simulink model "bd_ser_elect_cosim"  (Simulink 4.1.1)
settings: Solver=ode1  SolverMode=SingleTasking  StartTime=0.0  StopTime=max(cyc_mph(:,1))  FixedStep=1  MaxStep=1  RelTol=1e-3  AbsTol=1e-3
undefined symbols (not defined in the file): cs_lo_soc, cs_max_pwr, cs_max_pwr_fall_rate, cs_max_pwr_rise_rate, cs_min_pwr, ex_calc, fc_emis, fc_spd_scale, fc_trq_scale, time_step, vinf
libraries: lib_cosimulation x21, lib_controls x4, lib_wheel x2, lib_help x2, lib_transmission x2, simulink3 x1, lib_interactive x1, lib_drive_cycle x1, lib_exhaust x1, lib_fuel_converter x1, lib_vehicle x1
settings Model: LastModifiedBy=ssprik  SaveTime=off  SaveOutput=off  LimitDataPoints=off  UnconnectedLineMsg=none  RTWTemplateMakefile=grt_vc.tmf  ExtModeTrigMode=oneshot  ExtModeArmWhenConnect=off
settings Model: ModifiedComment=|
  | mokeefe -- Thu Apr 18 08:09:28 2002 -- Version 1.121
  | saving the model:
  | o "without the model browser open"
  | o with only top-level screen visible
  | o and with "fit to view" enabled
settings Model: ModifiedHistory=|
  | mokeefe -- Thu Apr 18 08:09:28 2002 -- Version 1.121
  | saving the model:
  | o "without the model browser open"
  | o with only top-level screen visible
  | o and with "fit to view" enabled

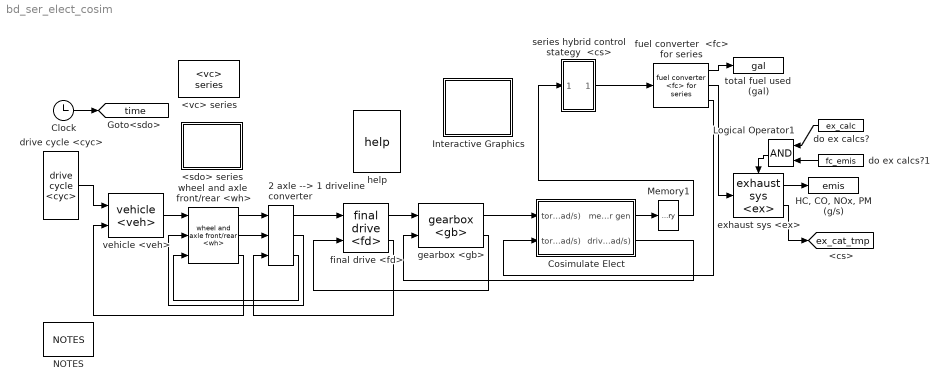
== system bd_ser_elect_cosim ==
  2 axle --> 1 driveline converter : lib_wheel/2 axle --> 1 driveline converter
      settings: RTWFcnNameOpts=Auto  RTWFileNameOpts=Auto
  <sdo> series : Subsystem
      settings: RTWFcnNameOpts=Auto  RTWFileNameOpts=Auto
      mask Display: image(imread('bdi_sdo.jpg'))
  <vc> series : lib_controls/<vc> series
      link override config traction control: BlockChoice=traction control
  Clock : Clock
      settings: DisplayTime=off  Decimation=10
  Cosimulate Elect : Subsystem  AncestorBlock=lib_cosimulation/SaberCosim
      settings: RTWFcnNameOpts=Auto  RTWFileNameOpts=Auto
      mask Display: image(imread('series_cosim.bmp'))
  "HC, CO, NOx, PM (g/s)" : ToWorkspace  VariableName=emis  SampleTime=0  SaveFormat=Array
  Interactive Graphics : Subsystem  BlockChoice=off
      link override off/Live Inputs/veh/roll res interactive: BlockChoice=roll res force req (N)
      settings: AttributesFormatString=%<BlockChoice>  TemplateBlock=lib_interactive/Interactive Graphics  MemberBlocks=off,on  RTWFcnNameOpts=Auto  RTWFileNameOpts=Auto
  Logical Operator1 : Logic  Orientation=left  Operator=AND  Inputs=2
  Memory1 : Memory  X0=0  InheritSampleTime=off
      settings: RTWStateStorageClass=Auto
  NOTES : lib_help/NOTES
  do ex calcs? : Constant  Orientation=left  Value=ex_calc
  do ex calcs?1 : Constant  Orientation=left  Value=fc_emis
  drive cycle <cyc> : lib_drive_cycle/drive cycle <cyc>
  exhaust sys <ex> : lib_exhaust/exhaust sys <ex>
  final drive <fd> : lib_transmission/final drive <fd>
  fuel converter  <fc> for series : lib_fuel_converter/fuel converter  <fc> for series
      link override fuel use and EO emis Configurable Subsystem: BlockChoice=fuel use and EO emis
  gearbox <gb> : lib_transmission/gearbox <gb>
  help : lib_help/help
  series hybrid control stategy  <cs> : Subsystem
      settings: RTWFcnNameOpts=Auto  RTWFileNameOpts=Auto
      mask Display: image(imread('bdi_cs.jpg'))
  total fuel used  (gal) : ToWorkspace  VariableName=gal  SampleTime=0  SaveFormat=Array
  vehicle <veh> : lib_vehicle/vehicle <veh>
      link override config force req'd to overcome rolling resistance: BlockChoice=force req'd to overcome rolling resistance (N)
      link override config vehicle speed: BlockChoice=vehicle speed (m/s)
      link override rolling resistance force: BlockChoice=force req'd to overcome rolling resistance (N)
      link override vehicle speed: BlockChoice=vehicle speed (m/s)
  wheel and axle  front/rear <wh> : lib_wheel/wheel and axle  front//rear <wh>
  tag scope: ex_cat_tmp=global, time=global
  wires:
  gearbox <gb>/1 -> Cosimulate Elect/1(torque and speed req'd at input side of gearbox (Nm),(rad/s))
  gearbox <gb>/2 -> final drive <fd>/2
  final drive <fd>/1 -> gearbox <gb>/1
  drive cycle <cyc>/1 -> vehicle <veh>/1
  Clock/1 -> [time]
  fuel converter  <fc> for series/2 -> exhaust sys <ex>/1
  fuel converter  <fc> for series/1 -> total fuel used  (gal)/1
  Logical Operator1/1 -> exhaust sys <ex>/Enable
  do ex calcs?/1 -> Logical Operator1/1
  exhaust sys <ex>/1 -> "HC, CO, NOx, PM (g/s)"/1
  do ex calcs?1/1 -> Logical Operator1/2
  exhaust sys <ex>/2 -> [ex_cat_tmp]
  fuel converter  <fc> for series/3 -> Cosimulate Elect/2(torque and speed available to drive line (Nm),(rad/s))
  Cosimulate Elect/2("drive torque and speed avail. at rotor (Nm), (rad/s)") -> gearbox <gb>/2
  Cosimulate Elect/1(mech pwr req'd for gen) -> Memory1/1
  Memory1/1 -> series hybrid control stategy  <cs>/1(mech power req'd from fc (W))
  series hybrid control stategy  <cs>/1("engine torque and speed (Nm), (rad/s)") -> fuel converter  <fc> for series/1
  vehicle <veh>/1 -> wheel and axle  front/rear <wh>/1
  wheel and axle  front/rear <wh>/1 -> 2 axle --> 1 driveline converter/1
  wheel and axle  front/rear <wh>/2 -> 2 axle --> 1 driveline converter/2
  2 axle --> 1 driveline converter/1 -> final drive <fd>/1
  2 axle --> 1 driveline converter/2 -> wheel and axle  front/rear <wh>/2
  2 axle --> 1 driveline converter/3 -> wheel and axle  front/rear <wh>/3
  final drive <fd>/2 -> 2 axle --> 1 driveline converter/3
  wheel and axle  front/rear <wh>/3 -> vehicle <veh>/2

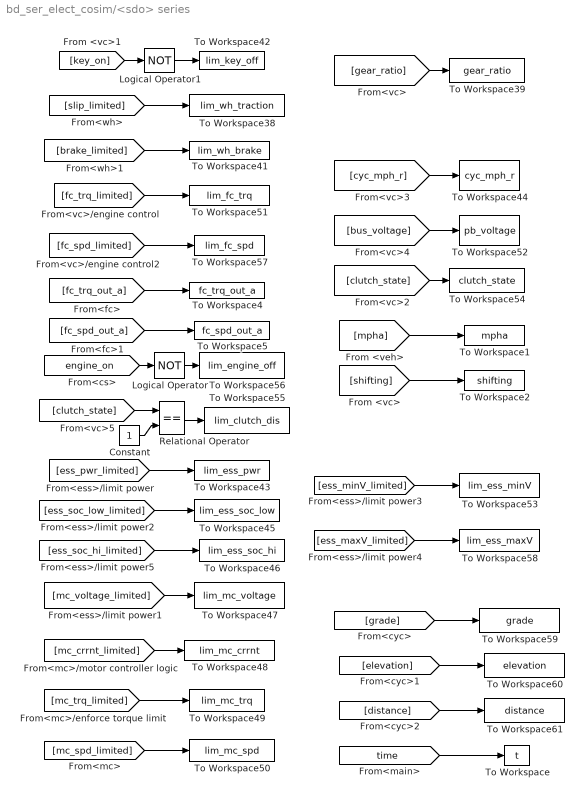
== system bd_ser_elect_cosim/<sdo> series ==
  Constant : Constant  Value=1
  Logical Operator : Logic  Operator=NOT  Inputs=1
  Logical Operator1 : Logic  Operator=NOT  Inputs=1
  Relational Operator : RelationalOperator  Operator===
  To Workspace : ToWorkspace  VariableName=t  SampleTime=0  SaveFormat=Array
  To Workspace1 : ToWorkspace  VariableName=mpha  SampleTime=-1  SaveFormat=Array
  To Workspace2 : ToWorkspace  VariableName=shifting  SampleTime=-1  SaveFormat=Array
  To Workspace38 : ToWorkspace  VariableName=lim_wh_traction  SampleTime=-1  SaveFormat=Array
  To Workspace39 : ToWorkspace  VariableName=gear_ratio  SampleTime=-1  SaveFormat=Array
  To Workspace4 : ToWorkspace  VariableName=fc_trq_out_a  SampleTime=-1  SaveFormat=Array
  To Workspace41 : ToWorkspace  VariableName=lim_wh_brake  SampleTime=-1  SaveFormat=Array
  To Workspace42 : ToWorkspace  VariableName=lim_key_off  SampleTime=-1  SaveFormat=Array
  To Workspace43 : ToWorkspace  VariableName=lim_ess_pwr  SampleTime=-1  SaveFormat=Array
  To Workspace44 : ToWorkspace  VariableName=cyc_mph_r  SampleTime=-1  SaveFormat=Array
  To Workspace45 : ToWorkspace  VariableName=lim_ess_soc_low  SampleTime=-1  SaveFormat=Array
  To Workspace46 : ToWorkspace  VariableName=lim_ess_soc_hi  SampleTime=-1  SaveFormat=Array
  To Workspace47 : ToWorkspace  VariableName=lim_mc_voltage  SampleTime=-1  SaveFormat=Array
  To Workspace48 : ToWorkspace  VariableName=lim_mc_crrnt  SampleTime=-1  SaveFormat=Array
  To Workspace49 : ToWorkspace  VariableName=lim_mc_trq  SampleTime=-1  SaveFormat=Array
  To Workspace5 : ToWorkspace  VariableName=fc_spd_out_a  SampleTime=-1  SaveFormat=Array
  To Workspace50 : ToWorkspace  VariableName=lim_mc_spd  SampleTime=-1  SaveFormat=Array
  To Workspace51 : ToWorkspace  VariableName=lim_fc_trq  SampleTime=-1  SaveFormat=Array
  To Workspace52 : ToWorkspace  VariableName=pb_voltage  SampleTime=-1  SaveFormat=Array
  To Workspace53 : ToWorkspace  VariableName=lim_ess_minV  SampleTime=-1  SaveFormat=Array
  To Workspace54 : ToWorkspace  VariableName=clutch_state  SampleTime=-1  SaveFormat=Array
  To Workspace55 : ToWorkspace  VariableName=lim_clutch_dis  SampleTime=-1  SaveFormat=Array
  To Workspace56 : ToWorkspace  VariableName=lim_engine_off  SampleTime=-1  SaveFormat=Array
  To Workspace57 : ToWorkspace  VariableName=lim_fc_spd  SampleTime=-1  SaveFormat=Array
  To Workspace58 : ToWorkspace  VariableName=lim_ess_maxV  SampleTime=-1  SaveFormat=Array
  To Workspace59 : ToWorkspace  VariableName=grade  SampleTime=-1  SaveFormat=Array
  To Workspace60 : ToWorkspace  VariableName=elevation  SampleTime=-1  SaveFormat=Array
  To Workspace61 : ToWorkspace  VariableName=distance  SampleTime=-1  SaveFormat=Array
  wires:
  [time] -> To Workspace/1
  [clutch_state] -> Relational Operator/1
  [fc_spd_out_a] -> To Workspace5/1
  [fc_trq_out_a] -> To Workspace4/1
  [mc_spd_limited] -> To Workspace50/1
  [mc_trq_limited] -> To Workspace49/1
  [mc_crrnt_limited] -> To Workspace48/1
  [mc_voltage_limited] -> To Workspace47/1
  [ess_soc_hi_limited] -> To Workspace46/1
  [ess_soc_low_limited] -> To Workspace45/1
  [ess_pwr_limited] -> To Workspace43/1
  Logical Operator/1 -> To Workspace56/1
  [engine_on] -> Logical Operator/1
  Constant/1 -> Relational Operator/2
  Relational Operator/1 -> To Workspace55/1
  [distance] -> To Workspace61/1
  [elevation] -> To Workspace60/1
  [grade] -> To Workspace59/1
  [ess_minV_limited] -> To Workspace53/1
  [ess_maxV_limited] -> To Workspace58/1
  Logical Operator1/1 -> To Workspace42/1
  [key_on] -> Logical Operator1/1
  [shifting] -> To Workspace2/1
  [mpha] -> To Workspace1/1
  [clutch_state] -> To Workspace54/1
  [bus_voltage] -> To Workspace52/1
  [cyc_mph_r] -> To Workspace44/1
  [gear_ratio] -> To Workspace39/1
  [slip_limited] -> To Workspace38/1
  [brake_limited] -> To Workspace41/1
  [fc_spd_limited] -> To Workspace57/1
  [fc_trq_limited] -> To Workspace51/1

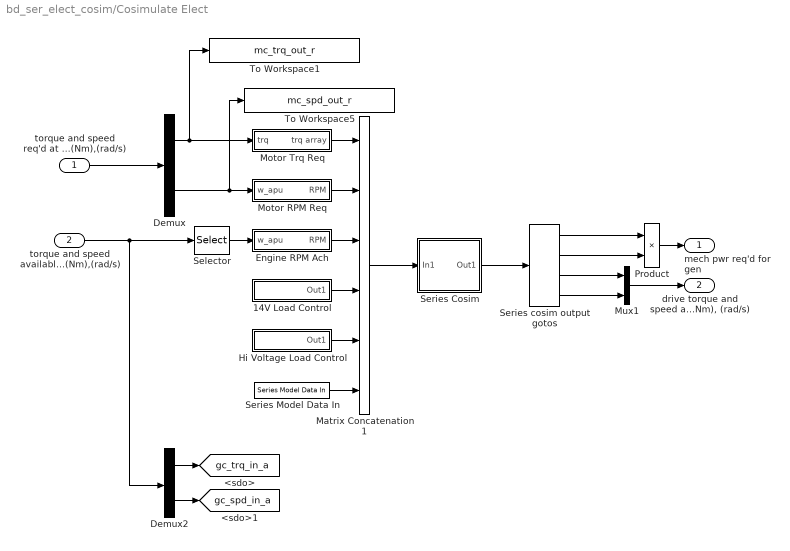
== system bd_ser_elect_cosim/Cosimulate Elect ==
  torque and speed req'd at input side of gearbox (Nm),(rad/s) : Inport  Port=1  LatchInput=off
  torque and speed available to drive line (Nm),(rad/s) : Inport  Port=2  LatchInput=off
  14V Load Control : Subsystem
      settings: RTWFcnNameOpts=Auto  RTWFileNameOpts=Auto
  Demux : Demux  Outputs=2  BusSelectionMode=off
  Demux2 : Demux  Outputs=2  BusSelectionMode=off
  Engine RPM Ach : Subsystem  AncestorBlock=lib_cosimulation/saber dv acc/Engine Info
      settings: RTWFcnNameOpts=Auto  RTWFileNameOpts=Auto
  Hi Voltage Load Control : Subsystem
      settings: RTWFcnNameOpts=Auto  RTWFileNameOpts=Auto
  Matrix Concatenation1 : simulink3/Signals & Systems/Matrix Concatenation  numInports=6  catMethod=Horizontal
  Motor RPM Req : Subsystem
      settings: RTWFcnNameOpts=Auto  RTWFileNameOpts=Auto
  Motor Trq Req : Subsystem
      settings: RTWFcnNameOpts=Auto  RTWFileNameOpts=Auto
  Mux1 : Mux  Inputs=2
  Product : Product  Inputs=2  Multiplication=Element-wise(.*)  SaturateOnIntegerOverflow=on
  Selector : Selector  InputType=Vector  ElementSrc=Internal  Elements=[2]  RowSrc=Internal  Rows=1  ColumnSrc=Internal  Columns=1  InputPortWidth=2
  Series Cosim : Subsystem  BlockChoice=Saber Text File Exchange
      settings: AttributesFormatString=%<BlockChoice>  TemplateBlock=lib_cosimulation/Series Cosim  MemberBlocks=Saber Text File Exchange,Series Saber Cosim,Series Simplorer Cosim  RTWFcnNameOpts=Auto  RTWFileNameOpts=Auto
  Series Model Data In : lib_cosimulation/Series Model Data In
  Series cosim output gotos : lib_cosimulation/Series cosim output gotos
      link override saber gc output gotos/Gain: Gain=1
      link override saber mc output gotos/sign convention: Gain=1
      settings: RTWFcnNameOpts=Auto  RTWFileNameOpts=Auto
  To Workspace1 : ToWorkspace  VariableName=mc_trq_out_r  SampleTime=-1  SaveFormat=Array
  To Workspace5 : ToWorkspace  VariableName=mc_spd_out_r  SampleTime=-1  SaveFormat=Array
  mech pwr req'd for gen : Outport  Port=1
  "drive torque and speed avail. at rotor (Nm), (rad/s)" : Outport  Port=2  InitialOutput=0
  tag scope: gc_spd_in_a=global, gc_trq_in_a=global
  wires:
  torque and speed req'd at input side of gearbox (Nm),(rad/s)/1 -> Demux/1
  Demux2/1 -> [gc_trq_in_a]
  Demux2/2 -> [gc_spd_in_a]
  Matrix Concatenation1/1 -> Series Cosim/1(In1)
  Series Cosim/1(Out1) -> Series cosim output gotos/1
  Mux1/1 -> "drive torque and speed avail. at rotor (Nm), (rad/s)"/1
  Series cosim output gotos/1 -> Product/1
  torque and speed available to drive line (Nm),(rad/s)/1 -> Selector/1, Demux2/1
  Demux/2 -> Motor RPM Req/1(w_apu), To Workspace5/1
  Motor RPM Req/1(RPM) -> Matrix Concatenation1/2
  Demux/1 -> Motor Trq Req/1(trq), To Workspace1/1
  Engine RPM Ach/1(RPM) -> Matrix Concatenation1/3
  Selector/1 -> Engine RPM Ach/1(w_apu)
  Motor Trq Req/1(trq array) -> Matrix Concatenation1/1
  Hi Voltage Load Control/1(Out1) -> Matrix Concatenation1/5
  14V Load Control/1(Out1) -> Matrix Concatenation1/4
  Series Model Data In/1 -> Matrix Concatenation1/6
  Series cosim output gotos/4 -> Mux1/2
  Series cosim output gotos/3 -> Mux1/1
  Series cosim output gotos/2 -> Product/2
  Product/1 -> mech pwr req'd for gen/1

== system bd_ser_elect_cosim/Interactive Graphics ==
  off : lib_interactive/off  Tag=Altia_off  Orientation=up

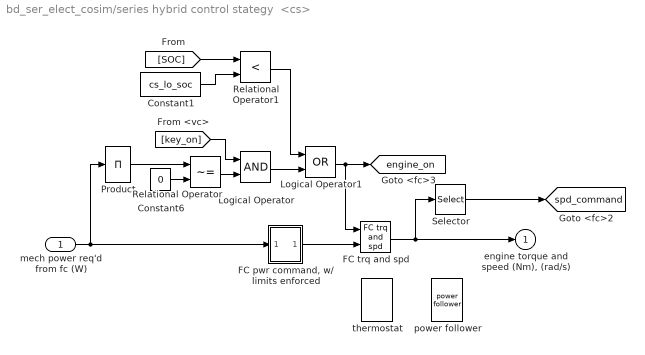
== system bd_ser_elect_cosim/series hybrid control stategy  <cs> ==
  mech power req'd from fc (W) : Inport  Port=1  LatchInput=off
  Constant1 : Constant  Value=cs_lo_soc
  Constant6 : Constant  Value=0
  "FC pwr command, w/ limits enforced" : Subsystem
      settings: RTWFcnNameOpts=Auto  RTWFileNameOpts=Auto
  FC trq and spd : lib_controls/series hybrid control stategy  <cs>/FC trq and spd
      settings: RTWFcnNameOpts=Auto  RTWFileNameOpts=Auto
  Logical Operator : Logic  Operator=AND  Inputs=2
  Logical Operator1 : Logic  Operator=OR  Inputs=2
  Product : Product  Inputs=1  Multiplication=Element-wise(.*)  SaturateOnIntegerOverflow=on
  Relational Operator : RelationalOperator  Operator=~=
  Relational Operator1 : RelationalOperator  Operator=<
  Selector : Selector  InputType=Vector  ElementSrc=Internal  Elements=2  RowSrc=Internal  Rows=1  ColumnSrc=Internal  Columns=1  InputPortWidth=2
  power follower : lib_controls/series hybrid control stategy  <cs>/power follower
  thermostat : lib_controls/series hybrid control stategy  <cs>/thermostat
  "engine torque and speed (Nm), (rad/s)" : Outport  Port=1  InitialOutput=0
  tag scope: engine_on=global, spd_command=global
  wires:
  Selector/1 -> [spd_command]
  mech power req'd from fc (W)/1 -> Product/1, "FC pwr command, w/ limits enforced"/1(FC pwr command)
  Constant6/1 -> Relational Operator/2
  Relational Operator/1 -> Logical Operator/2
  [key_on] -> Logical Operator/1
  Product/1 -> Relational Operator/1
  "FC pwr command, w/ limits enforced"/1(limited FC pwr command (W)) -> FC trq and spd/2
  FC trq and spd/1 -> "engine torque and speed (Nm), (rad/s)"/1, Selector/1
  Logical Operator1/1 -> [engine_on], FC trq and spd/1
  Logical Operator/1 -> Logical Operator1/2
  [SOC] -> Relational Operator1/1
  Constant1/1 -> Relational Operator1/2
  Relational Operator1/1 -> Logical Operator1/1

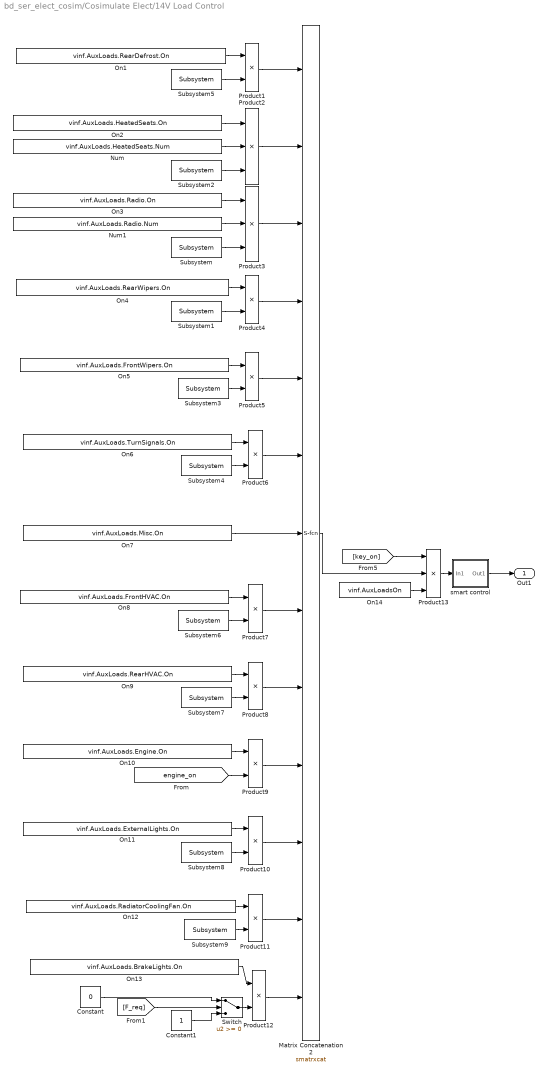
== system bd_ser_elect_cosim/Cosimulate Elect/14V Load Control ==
  Constant : Constant  Value=0
  Constant1 : Constant  Value=1
  Matrix Concatenation2 : S-Function  FunctionName=smatrxcat  Parameters=numInports,catMethod  PortCounts=[]  SFunctionModules=''  mask(Matrix Concatenation){numInports=13, catMethod=Horizontal}
      mask prompts: numInports "Number of inputs:"; catMethod "Concatenation method:"
      mask help: Perform horizontal or vertical concatenation. 1-D vector input signals are treated as column vectors, i.e., [Mx1] matrices. The output is always a matrix.
      mask init:
      | xy = matrxcatmask('icon');
      mask StyleString: edit,popup(Horizontal|Vertical)
      mask Display:
      | plot(xy.x,xy.y);
      | text(0.15,0.86,xy.label);
  Num : Constant  Value=vinf.AuxLoads.HeatedSeats.Num
  Num1 : Constant  Value=vinf.AuxLoads.Radio.Num
  On1 : Constant  Value=vinf.AuxLoads.RearDefrost.On
  On10 : Constant  Value=vinf.AuxLoads.Engine.On
  On11 : Constant  Value=vinf.AuxLoads.ExternalLights.On
  On12 : Constant  Value=vinf.AuxLoads.RadiatorCoolingFan.On
  On13 : Constant  Value=vinf.AuxLoads.BrakeLights.On
  On14 : Constant  Value=vinf.AuxLoadsOn
  On2 : Constant  Value=vinf.AuxLoads.HeatedSeats.On
  On3 : Constant  Value=vinf.AuxLoads.Radio.On
  On4 : Constant  Value=vinf.AuxLoads.RearWipers.On
  On5 : Constant  Value=vinf.AuxLoads.FrontWipers.On
  On6 : Constant  Value=vinf.AuxLoads.TurnSignals.On
  On7 : Constant  Value=vinf.AuxLoads.Misc.On
  On8 : Constant  Value=vinf.AuxLoads.FrontHVAC.On
  On9 : Constant  Value=vinf.AuxLoads.RearHVAC.On
  Product{1,4..12} (10 alike) : Product  Inputs=2  Multiplication=Element-wise(.*)  SaturateOnIntegerOverflow=on
  Product13 : Product  Inputs=3  Multiplication=Element-wise(.*)  SaturateOnIntegerOverflow=on
  Product2 : Product  Inputs=3  Multiplication=Element-wise(.*)  SaturateOnIntegerOverflow=on
  Product3 : Product  Inputs=3  Multiplication=Element-wise(.*)  SaturateOnIntegerOverflow=on
  Subsystem : lib_cosimulation/Subsystem  ModelName='Radio'
  Subsystem1 : lib_cosimulation/Subsystem  ModelName='RearWipers'
  Subsystem2 : lib_cosimulation/Subsystem  ModelName='HeatedSeats'
  Subsystem3 : lib_cosimulation/Subsystem  ModelName='FrontWipers'
  Subsystem4 : lib_cosimulation/Subsystem  ModelName='TurnSignals'
  Subsystem5 : lib_cosimulation/Subsystem  ModelName='RearDefrost'
  Subsystem6 : lib_cosimulation/Subsystem  ModelName='FrontHVAC'
  Subsystem7 : lib_cosimulation/Subsystem  ModelName='RearHVAC'
  Subsystem8 : lib_cosimulation/Subsystem  ModelName='ExternalLights'
  Subsystem9 : lib_cosimulation/Subsystem  ModelName='RadiatorCoolingFan'
  Switch : Switch  Threshold=0
  smart control : Subsystem
      settings: RTWFcnNameOpts=Auto  RTWFileNameOpts=Auto
  Out1 : Outport  Port=1
  wires:
  Subsystem/1 -> Product3/3
  Product1/1 -> Matrix Concatenation2/1
  smart control/1(Out1) -> Out1/1
  On14/1 -> Product13/3
  Subsystem5/1 -> Product1/2
  On1/1 -> Product1/1
  Subsystem2/1 -> Product2/3
  Num/1 -> Product2/2
  On2/1 -> Product2/1
  Num1/1 -> Product3/2
  On3/1 -> Product3/1
  Subsystem1/1 -> Product4/2
  On4/1 -> Product4/1
  Subsystem3/1 -> Product5/2
  On5/1 -> Product5/1
  On6/1 -> Product6/1
  Subsystem4/1 -> Product6/2
  On7/1 -> Matrix Concatenation2/7
  Subsystem6/1 -> Product7/2
  On8/1 -> Product7/1
  Subsystem7/1 -> Product8/2
  [engine_on] -> Product9/2
  On10/1 -> Product9/1
  Subsystem8/1 -> Product10/2
  On11/1 -> Product10/1
  Subsystem9/1 -> Product11/2
  On12/1 -> Product11/1
  Switch/1 -> Product12/2
  Constant1/1 -> Switch/3
  [F_req] -> Switch/2
  Constant/1 -> Switch/1
  On13/1 -> Product12/1
  Product2/1 -> Matrix Concatenation2/2
  Product3/1 -> Matrix Concatenation2/3
  Product4/1 -> Matrix Concatenation2/4
  Product5/1 -> Matrix Concatenation2/5
  Product6/1 -> Matrix Concatenation2/6
  Product7/1 -> Matrix Concatenation2/8
  Product8/1 -> Matrix Concatenation2/9
  Product9/1 -> Matrix Concatenation2/10
  Product10/1 -> Matrix Concatenation2/11
  Product11/1 -> Matrix Concatenation2/12
  Product12/1 -> Matrix Concatenation2/13
  On9/1 -> Product8/1
  Product13/1 -> smart control/1(In1)
  [key_on] -> Product13/1
  Matrix Concatenation2/1 -> Product13/2

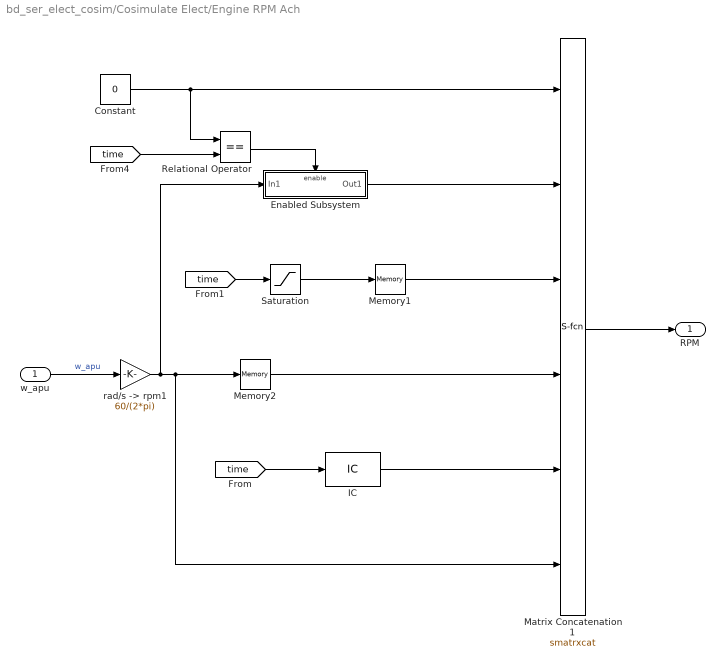
== system bd_ser_elect_cosim/Cosimulate Elect/Engine RPM Ach ==
  w_apu : Inport  Port=1  LatchInput=off
  Constant : Constant  Value=0
  Enabled Subsystem : Subsystem  TreatAsAtomicUnit=on
      settings: RTWFcnNameOpts=Auto  RTWFileNameOpts=Auto
  IC : InitialCondition  Value=time_step
  Matrix Concatenation1 : S-Function  FunctionName=smatrxcat  Parameters=numInports,catMethod  PortCounts=[]  SFunctionModules=''  mask(Matrix Concatenation){numInports=6, catMethod=Horizontal}
      mask prompts: numInports "Number of inputs:"; catMethod "Concatenation method:"
      mask help: Perform horizontal or vertical concatenation. 1-D vector input signals are treated as column vectors, i.e., [Mx1] matrices. The output is always a matrix.
      mask init:
      | xy = matrxcatmask('icon');
      mask StyleString: edit,popup(Horizontal|Vertical)
      mask Display:
      | plot(xy.x,xy.y);
      | text(0.15,0.86,xy.label);
  Memory1 : Memory  X0=.001  InheritSampleTime=on
      settings: RTWStateStorageClass=Auto
  Memory2 : Memory  X0=80  InheritSampleTime=on
      settings: RTWStateStorageClass=Auto
  Relational Operator : RelationalOperator  Operator===
  Saturation : Saturate  UpperLimit=inf  LowerLimit=.001  LinearizeAsGain=on
  "rad/s -> rpm1" : Gain  Gain=60/(2*pi)  Multiplication=Element-wise(K.*u)  SaturateOnIntegerOverflow=on
  RPM : Outport  Port=1
  wires:
  Relational Operator/1 -> Enabled Subsystem/Enable
  [time] -> Relational Operator/2
  Enabled Subsystem/1(Out1) -> Matrix Concatenation1/2
  Memory2/1 -> Matrix Concatenation1/4
  Matrix Concatenation1/1 -> RPM/1
  IC/1 -> Matrix Concatenation1/5
  Saturation/1 -> Memory1/1
  [time] -> Saturation/1
  Memory1/1 -> Matrix Concatenation1/3
  [time] -> IC/1
  Constant/1 -> Relational Operator/1, Matrix Concatenation1/1
  w_apu/1 -> "rad/s -> rpm1"/1  "w_apu"
  "rad/s -> rpm1"/1 -> Memory2/1, Matrix Concatenation1/6, Enabled Subsystem/1(In1)

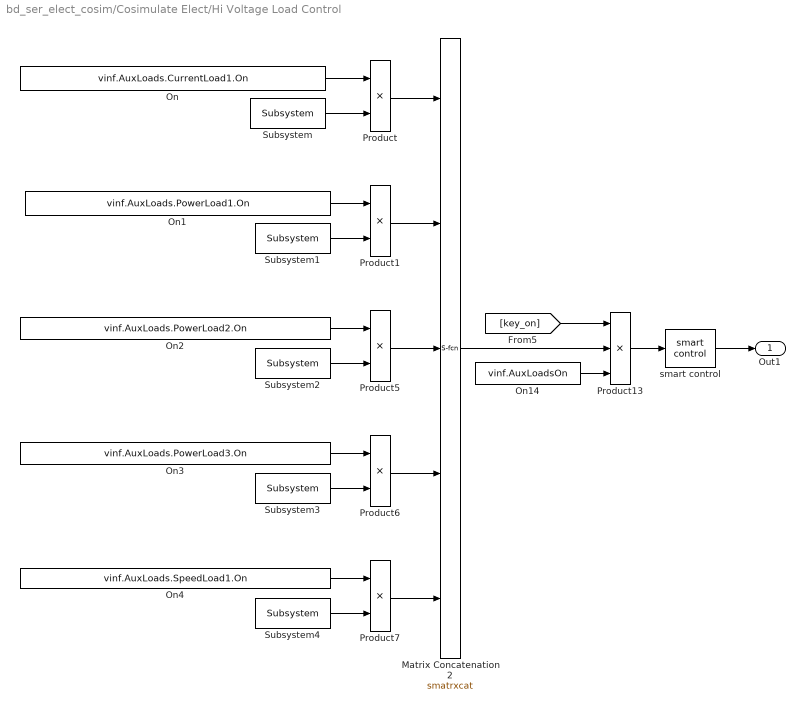
== system bd_ser_elect_cosim/Cosimulate Elect/Hi Voltage Load Control ==
  Matrix Concatenation2 : S-Function  FunctionName=smatrxcat  Parameters=numInports,catMethod  PortCounts=[]  SFunctionModules=''  mask(Matrix Concatenation){numInports=5, catMethod=Horizontal}
      mask prompts: numInports "Number of inputs:"; catMethod "Concatenation method:"
      mask help: Perform horizontal or vertical concatenation. 1-D vector input signals are treated as column vectors, i.e., [Mx1] matrices. The output is always a matrix.
      mask init:
      | xy = matrxcatmask('icon');
      mask StyleString: edit,popup(Horizontal|Vertical)
      mask Display:
      | plot(xy.x,xy.y);
      | text(0.15,0.86,xy.label);
  On : Constant  Value=vinf.AuxLoads.CurrentLoad1.On
  On1 : Constant  Value=vinf.AuxLoads.PowerLoad1.On
  On14 : Constant  Value=vinf.AuxLoadsOn
  On2 : Constant  Value=vinf.AuxLoads.PowerLoad2.On
  On3 : Constant  Value=vinf.AuxLoads.PowerLoad3.On
  On4 : Constant  Value=vinf.AuxLoads.SpeedLoad1.On
  Product{,1,5..7} (5 alike) : Product  Inputs=2  Multiplication=Element-wise(.*)  SaturateOnIntegerOverflow=on
  Product13 : Product  Inputs=3  Multiplication=Element-wise(.*)  SaturateOnIntegerOverflow=on
  Subsystem : lib_cosimulation/Subsystem  ModelName='CurrentLoad1'
  Subsystem1 : lib_cosimulation/Subsystem  ModelName='PowerLoad1'
  Subsystem2 : lib_cosimulation/Subsystem  ModelName='PowerLoad2'
  Subsystem3 : lib_cosimulation/Subsystem  ModelName='PowerLoad3'
  Subsystem4 : lib_cosimulation/Subsystem  ModelName='SpeedLoad1'
  smart control : lib_cosimulation/14V Load Control/smart control
      settings: RTWFcnNameOpts=Auto  RTWFileNameOpts=Auto
  Out1 : Outport  Port=1
  wires:
  smart control/1 -> Out1/1
  On14/1 -> Product13/3
  [key_on] -> Product13/1
  Product13/1 -> smart control/1
  Subsystem/1 -> Product/2
  On/1 -> Product/1
  Product/1 -> Matrix Concatenation2/1
  Subsystem2/1 -> Product5/2
  On2/1 -> Product5/1
  Subsystem3/1 -> Product6/2
  On3/1 -> Product6/1
  On4/1 -> Product7/1
  Subsystem4/1 -> Product7/2
  Product1/1 -> Matrix Concatenation2/2
  Product5/1 -> Matrix Concatenation2/3
  Product6/1 -> Matrix Concatenation2/4
  Product7/1 -> Matrix Concatenation2/5
  Subsystem1/1 -> Product1/2
  On1/1 -> Product1/1
  Matrix Concatenation2/1 -> Product13/2

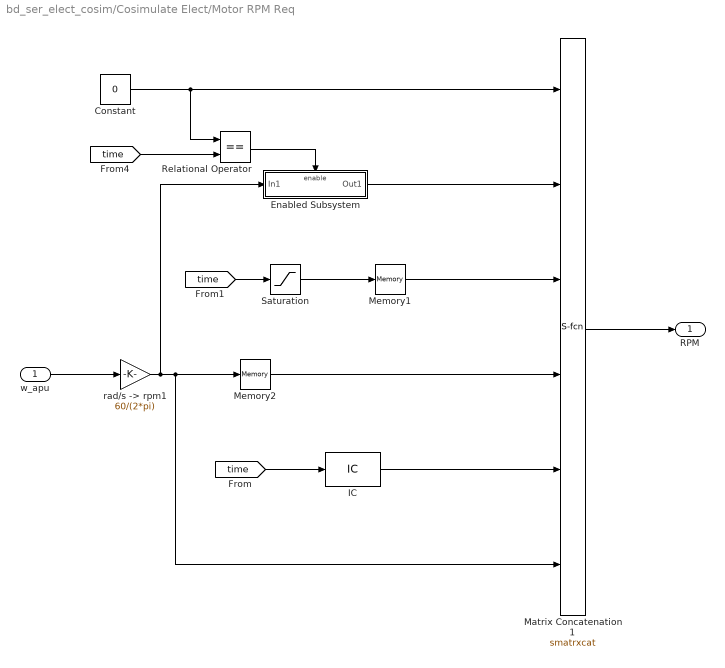
== system bd_ser_elect_cosim/Cosimulate Elect/Motor RPM Req ==
  w_apu : Inport  Port=1  LatchInput=off
  Constant : Constant  Value=0
  Enabled Subsystem : Subsystem  TreatAsAtomicUnit=on
      settings: RTWFcnNameOpts=Auto  RTWFileNameOpts=Auto
  IC : InitialCondition  Value=time_step
  Matrix Concatenation1 : S-Function  FunctionName=smatrxcat  Parameters=numInports,catMethod  PortCounts=[]  SFunctionModules=''  mask(Matrix Concatenation){numInports=6, catMethod=Horizontal}
      mask prompts: numInports "Number of inputs:"; catMethod "Concatenation method:"
      mask help: Perform horizontal or vertical concatenation. 1-D vector input signals are treated as column vectors, i.e., [Mx1] matrices. The output is always a matrix.
      mask init:
      | xy = matrxcatmask('icon');
      mask StyleString: edit,popup(Horizontal|Vertical)
      mask Display:
      | plot(xy.x,xy.y);
      | text(0.15,0.86,xy.label);
  Memory1 : Memory  X0=.001  InheritSampleTime=on
      settings: RTWStateStorageClass=Auto
  Memory2 : Memory  X0=0  InheritSampleTime=on
      settings: RTWStateStorageClass=Auto
  Relational Operator : RelationalOperator  Operator===
  Saturation : Saturate  UpperLimit=inf  LowerLimit=.001  LinearizeAsGain=on
  "rad/s -> rpm1" : Gain  Gain=60/(2*pi)  Multiplication=Element-wise(K.*u)  SaturateOnIntegerOverflow=on
  RPM : Outport  Port=1
  wires:
  Relational Operator/1 -> Enabled Subsystem/Enable
  [time] -> Relational Operator/2
  Enabled Subsystem/1(Out1) -> Matrix Concatenation1/2
  Memory2/1 -> Matrix Concatenation1/4
  Matrix Concatenation1/1 -> RPM/1
  IC/1 -> Matrix Concatenation1/5
  Saturation/1 -> Memory1/1
  [time] -> Saturation/1
  Memory1/1 -> Matrix Concatenation1/3
  [time] -> IC/1
  Constant/1 -> Relational Operator/1, Matrix Concatenation1/1
  w_apu/1 -> "rad/s -> rpm1"/1
  "rad/s -> rpm1"/1 -> Memory2/1, Matrix Concatenation1/6, Enabled Subsystem/1(In1)

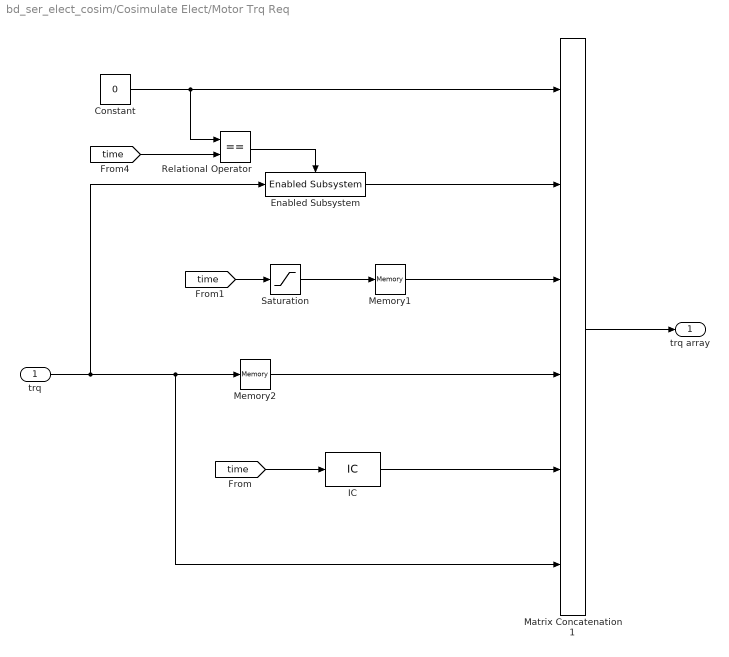
== system bd_ser_elect_cosim/Cosimulate Elect/Motor Trq Req ==
  trq : Inport  Port=1  LatchInput=off
  Constant : Constant  Value=0
  Enabled Subsystem : lib_cosimulation/saber dv acc/Engine Info/Enabled Subsystem  TreatAsAtomicUnit=on
      settings: RTWFcnNameOpts=Auto  RTWFileNameOpts=Auto
  IC : InitialCondition  Value=time_step
  Matrix Concatenation1 : lib_cosimulation/saber dv acc/Engine Info/Matrix Concatenation1  numInports=6  catMethod=Horizontal
  Memory1 : Memory  X0=.001  InheritSampleTime=on
      settings: RTWStateStorageClass=Auto
  Memory2 : Memory  X0=0  InheritSampleTime=on
      settings: RTWStateStorageClass=Auto
  Relational Operator : RelationalOperator  Operator===
  Saturation : Saturate  UpperLimit=inf  LowerLimit=.001  LinearizeAsGain=on
  trq array : Outport  Port=1
  wires:
  trq/1 -> Enabled Subsystem/1, Memory2/1, Matrix Concatenation1/6
  Constant/1 -> Matrix Concatenation1/1, Relational Operator/1
  [time] -> IC/1
  Memory1/1 -> Matrix Concatenation1/3
  [time] -> Saturation/1
  Saturation/1 -> Memory1/1
  IC/1 -> Matrix Concatenation1/5
  Matrix Concatenation1/1 -> trq array/1
  Memory2/1 -> Matrix Concatenation1/4
  Enabled Subsystem/1 -> Matrix Concatenation1/2
  [time] -> Relational Operator/2
  Relational Operator/1 -> Enabled Subsystem/Enable

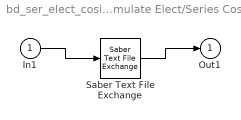
== system bd_ser_elect_cosim/Cosimulate Elect/Series Cosim ==
  In1 : Inport  Port=1  LatchInput=off
  Saber Text File Exchange : lib_cosimulation/Saber Text File Exchange  AncestorBlock=lib_cosimulation/SaberCosim
  Out1 : Outport  Port=1
  wires:
  In1/1 -> Saber Text File Exchange/1
  Saber Text File Exchange/1 -> Out1/1

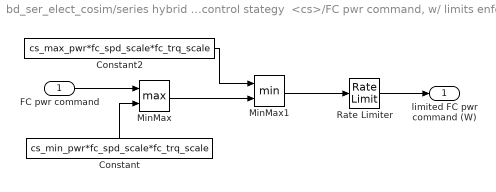
== system bd_ser_elect_cosim/series hybrid control stategy  <cs>/FC pwr command, w/ limits enforced ==
  FC pwr command : Inport  Port=1  LatchInput=off
  Constant : Constant  Orientation=up  Value=cs_min_pwr*fc_spd_scale*fc_trq_scale
  Constant2 : Constant  Value=cs_max_pwr*fc_spd_scale*fc_trq_scale
  MinMax : MinMax  Function=max  Inputs=2
  MinMax1 : MinMax  Function=min  Inputs=2
  Rate Limiter : RateLimiter  RisingSlewLimit=cs_max_pwr_rise_rate*fc_spd_scale*fc_trq_scale  FallingSlewLimit=cs_max_pwr_fall_rate*fc_spd_scale*fc_trq_scale
  limited FC pwr command (W) : Outport  Port=1
  wires:
  FC pwr command/1 -> MinMax/1
  MinMax/1 -> MinMax1/2
  Constant/1 -> MinMax/2
  Rate Limiter/1 -> limited FC pwr command (W)/1
  MinMax1/1 -> Rate Limiter/1
  Constant2/1 -> MinMax1/1

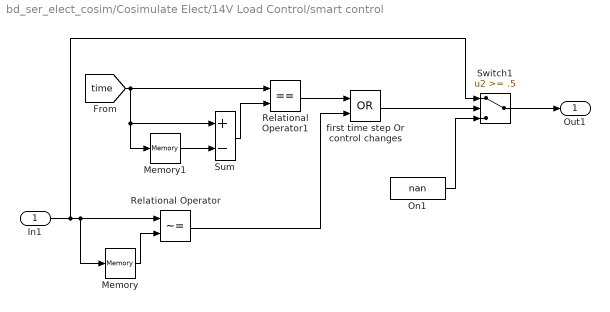
== system bd_ser_elect_cosim/Cosimulate Elect/14V Load Control/smart control ==
  In1 : Inport  Port=1  LatchInput=off
  Memory : Memory  X0=0  InheritSampleTime=off
      settings: RTWStateStorageClass=Auto
  Memory1 : Memory  X0=0  InheritSampleTime=off
      settings: RTWStateStorageClass=Auto
  On1 : Constant  Value=nan
  Relational Operator : RelationalOperator  Operator=~=
  Relational Operator1 : RelationalOperator  Operator===
  Sum : Sum  Inputs=+-  SaturateOnIntegerOverflow=on
  Switch1 : Switch  Threshold=.5
  first time step Or control changes : Logic  Operator=OR  Inputs=2
  Out1 : Outport  Port=1
  wires:
  Memory1/1 -> Sum/2
  On1/1 -> Switch1/3
  Switch1/1 -> Out1/1
  Relational Operator/1 -> first time step Or control changes/2
  Sum/1 -> Relational Operator1/2
  Relational Operator1/1 -> first time step Or control changes/1
  first time step Or control changes/1 -> Switch1/2
  [time] -> Memory1/1, Sum/1, Relational Operator1/1
  Memory/1 -> Relational Operator/2
  In1/1 -> Switch1/1, Relational Operator/1, Memory/1

== system bd_ser_elect_cosim/Cosimulate Elect/Engine RPM Ach/Enabled Subsystem ==
  In1 : Inport  Port=1  LatchInput=off
  Enable : EnablePort
  Out1 : Outport  Port=1
  wires:
  In1/1 -> Out1/1

== system bd_ser_elect_cosim/Cosimulate Elect/Motor RPM Req/Enabled Subsystem ==
  In1 : Inport  Port=1  LatchInput=off
  Enable : EnablePort
  Out1 : Outport  Port=1
  wires:
  In1/1 -> Out1/1
